simulink model "rest_api_task"  (Simulink 3.00)
libraries: mathlib x5, stringlib x1, arclib x1

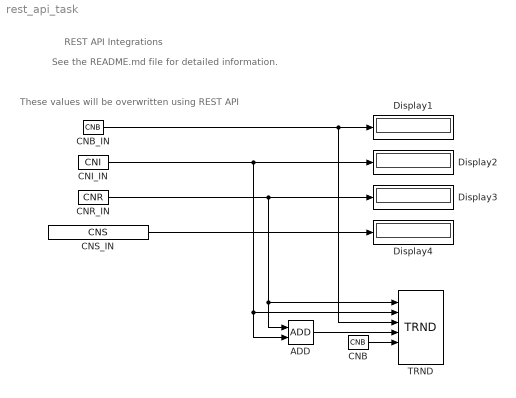
== system rest_api_task ==
  note: See the README.md file for detailed information.
  note: REST API Integrations
  note: These values will be overwritten
      | using REST API
  ADD : mathlib/ADD
  CNB : mathlib/CNB  YCN=on
  CNB_IN : mathlib/CNB  YCN=off
  CNI_IN : mathlib/CNI  icn=7
  CNR_IN : mathlib/CNR  ycn=12.3
  CNS_IN : stringlib/CNS  scv=My string  nmax=0
  Display{1..4} (4 alike) : Display
      settings: Format=Best fit
  TRND : arclib/TRND  n=4  l=5000  btype=8: Double  ptype1=1: Store  ptype2=1: Store  ptype3=1: Store  ptype4=1: Store  pfac=1  afac=0  arc=0  id=0  Title=Values in time  timesrc=1: CORETIMER
  wires:
  ADD/1 -> TRND/4
  CNB/1 -> TRND/5
  CNB_IN/1 -> Display1/1, TRND/3
  CNI_IN/1 -> Display2/1, ADD/2, TRND/2
  CNR_IN/1 -> Display3/1, ADD/1, TRND/1
  CNS_IN/1 -> Display4/1
